simulink model "Solver"  (R2016b)
settings: Solver=ode4  StartTime=0.0  StopTime=Inf  FixedStep=base_dT  RelTol=1e-3
values from neighbouring files (symbols this model uses):
  base_dT = Simulink.Parameter    [SolverInit.m]
  E2C_bEgoFol = Simulink.Parameter    [SolverInit.m]
  E2C_bUseCollo = Simulink.Parameter    [SolverInit.m]
  E2C_c2_dTB = Simulink.Parameter    [SolverInit.m]
  E2C_c_dTB = Simulink.Parameter    [SolverInit.m]
  E2C_d_HDW1 = Simulink.Parameter    [SolverInit.m]
  E2C_d_HDW2 = Simulink.Parameter    [SolverInit.m]
  E2C_DeltaT = Simulink.Parameter    [SolverInit.m]
  E2C_df_term = Simulink.Parameter    [SolverInit.m]
  E2C_dz_term = Simulink.Parameter    [SolverInit.m]
  E2C_Max_iter = Simulink.Parameter    [SolverInit.m]
  E2C_t_HDW1 = Simulink.Parameter    [SolverInit.m]
  E2C_t_HDW2 = Simulink.Parameter    [SolverInit.m]
  E2C_T_TB_thr = Simulink.Parameter    [SolverInit.m]
  E2C_tiSolverPeriod_C = Simulink.Parameter    [SolverInit.m]
  E2C_U_max = Simulink.Parameter    [SolverInit.m]
  E2C_U_min = Simulink.Parameter    [SolverInit.m]
  E2C_V_max = Simulink.Parameter    [SolverInit.m]
  E2C_V_min = Simulink.Parameter    [SolverInit.m]
  E2C_w_delta_u = Simulink.Parameter    [SolverInit.m]
  E2C_w_epsilon_lin = Simulink.Parameter    [SolverInit.m]
  E2C_weight_TTB = Simulink.Parameter    [SolverInit.m]
  Inp_mf_exh_par = Simulink.Parameter    [SolverInit.m]
  Inp_t_eu_par = Simulink.Parameter    [SolverInit.m]
  NP_trial = Simulink.Parameter    [SolverInit.m]
  t_EndSimulation = Simulink.Parameter    [SolverInit.m]
  t_StartSimulation = Simulink.Parameter    [SolverInit.m]
libraries: simulink x3, dspsigops x2
(part 1 of 2)
settings Model: Creator=Tulga Ersal  LastModifiedBy=Hcn
settings OptimizationCC: BlockReduction=off  BooleanDataType=off  LifeSpan=inf
settings DebuggingCC: SaveWithParameterizedLinksMsg=none  UnderspecifiedInitializationDetection=Classic  MergeDetectMultiDrivingBlocksExec=none  SignalResolutionControl=TryResolveAllWithWarning  SFUnexpectedBacktrackingDiag=warning  SFNoUnconditionalDefaultTransitionDiag=warning  SFExecutionAtInitializationDiag=none
settings HardwareCC: TargetBitPerPointer=64  TargetBitPerSizeT=64  TargetBitPerPtrDiffT=64  TargetLongLongMode=on  TargetIntDivRoundTo=Zero  TargetEndianess=LittleEndian  TargetWordSize=64  TargetHWDeviceType=MATLAB Host  ProdEqTarget=off
settings ModelReferenceCC: PropagateSignalLabelsOutOfModel=off
settings GRTTargetCC: TargetLangStandard=C89/C90 (ANSI)
settings ConfigComp: CovMetricSettings=dw  CovHtmlReporting=on  CovSaveCumulativeToWorkspaceVar=on  CovSaveSingleToWorkspaceVar=on  CovExternalEMLEnable=off

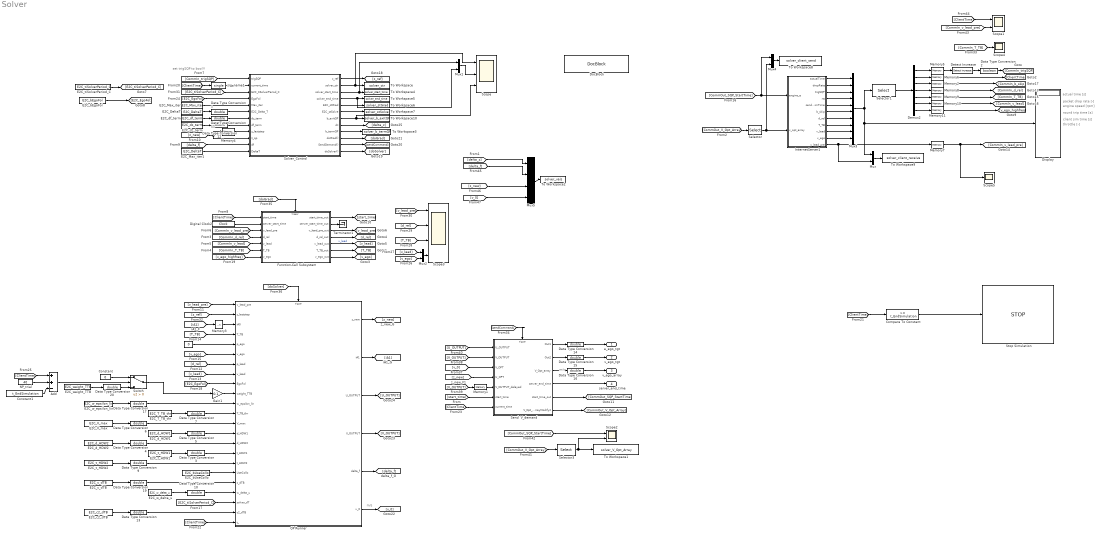
== system Solver ==
  note: set trigSQP to bool!!
  note: packet drop rate [-]
  note: actual time [s]
  note: engine speed [rpm]
  note: round trip time [s]
  note: client sim time [s]
  note: throttle [-]
  note: m/s
  note: m/s
  "\t" : Constant  Value=0
  Add : Sum  Inputs=++-
  Compare To Constant : simulink/Logic and Bit Operations/Compare To Constant  relop=>=  const=t_EndSimulation  OutDataTypeStr=boolean
  Constant : Constant  Value=0
  Constant1 : Constant  Value=t_EndSimulation
  Data Type Conversion{1,3..7,9..17,19..20} (17 alike) : DataTypeConversion  OutDataTypeStr=double
  Data Type Conversion2 : DataTypeConversion  OutDataTypeStr=boolean
  Demux2 : Demux  Outputs=7
  Detect Increase : simulink/Logic and Bit Operations/Detect Increase  vinit=0.0  OutDataTypeStr=boolean
  Digital Clock2 : DigitalClock  SampleTime=base_dT
  Display : Display
  DocBlock : simulink/Model-Wide Utilities/DocBlock  DocumentType=Text
      content=|
      | 110719T1200         -Finish chart for customized process control
      | 110719T1500         -use Ts=0.1(hardcoded), run server model alone, process control works with EgoFol=1.
      | 110719T1630         -use Ts=base_dT=0.01, run server & client. EgoFol=1.
      | 111119T1200         -Use last_v_opt(solver_start-delayed(solver_start) ) as current v_ego_tgt.
      |                     -Put the modification in Send V_demand subsys.
      |                     -Avoid using another block with detectchange in solver_end_time to trigger this modification.
      |                     -Clean the model and setup communication input/output ports (magenta)
      |                     -Modify Solver_Control so that EgoFol=0 case also works
      | 111119T2200         -Comment out "simulink execution control"
      |                     -If at one step "solver_exec_time>1s", the delay will cumulate
      |                     -need logic control in client to decide whether to skip a trigger.
      | 111219T1300         -Use Client time to set b_termQP.
      |                     -Set E2C_DeltaT=0.3s, save 0.3s for communication
      |                     -Cannot reset if one communication takes long time.
      | Client_112619T1415  -Created from PlatoonModel_Chunan_2016b_112119T1155 and InternetClient_112619T1300.
      |                     -Contains the whole vehicle model.
      |                     -Set up memory for CommOut_V_Opt_Array to align change for CommOut_V_Opt_Array and Comm_Start_Time.
      | Solver_112619T1415  -Created.
      |                     -Add semicolon in state flow to avoid printing intermediate variables.
      | Solver_112719T1142  -Add solver_ctr to workspace
      |                     -Do 10 "dosolver" in 1 step to compensate for base_dT=0.1s. If base_dT=0.01, use 1 dosolver.
      | Solver_112719T2200  -PlatoonModel_Chunan_2016b_112719T2200_solver/Send  V_demand/Triggered Subsystem.
      |                     Change also ceil(current_time-last_start_time).
      | C/S_122019T1424     -Add to resolve rtt issue. Not very useful on full model.:
      |                             while (myIns.simTime > timeNow*1)
      |                          {
      |                              QueryPerformanceCounter(&LItNow);
      |                              timeNow = ((double)(LItNow.QuadPart - G.LIstartTime.QuadPart)) / ((double)(G.LIticksPerSecond.QuadPart)) ;
      |                          }
      | C+S_122019T1618     -Put original solver and client into one system.
      |                     -Now the sent information are place holders to maintain dimension.
      |                     -Finally if this works, the client will be BBK and only sends
      |                     torque, TTB. Solver sends Ne, Alpha.
      | S_122819T1229 (C_122019T1618)
      |                     -Apply changes from Tulga in email "reducing delay further" to 122019T1618.
      |                     -rrt maintains to be 0.02s = base_dT.
      | S_122819T1301 (C_122019T1424)
      |                     -Apply changes from Tulga in email "reducing delay further" to 122019T1424.
      |                     -rrt drops to 0.02s = base_dT.
      |                     -But optimization result is still bad.
      |                     Does not recover optimal results similar to platoonmodel(without interenet),
      |                     like in version S_122819T1229.
      |                     -(!!!)switch Commin_v_lead and v_ego_highfreq at output of InternetServer1 demux.
      | %%%%%%%%%%%%%%%%%%%%%%%%%%%%%%%%%%%%%%%%%%%%%%%%%%%%%%%%%%%%%%%%%%%%%%%%%%
      | %                        3-computer setup                                %
      | %%%%%%%%%%%%%%%%%%%%%%%%%%%%%%%%%%%%%%%%%%%%%%%%%%%%%%%%%%%%%%%%%%%%%%%%%%
      | Solver_01022020T1343
      |                     -Create "InternetSolverInit.m" file for initialization.
      |                     -Only need "SpeedAcceMap8.mat" as external datasource.
  E2C_DeltaT : Constant  Value=E2C_DeltaT  OutDataTypeStr=double
  E2C_Max_iter : Constant  Value=E2C_Max_iter  OutDataTypeStr=int8
  E2C_Max_iter1 : Constant  Value=E2C_DeltaT  OutDataTypeStr=single
  E2C_T_TB_thr : Constant  Value=E2C_T_TB_thr  OutDataTypeStr=double
  E2C_V_max : Constant  Value=E2C_V_max  OutDataTypeStr=double
  E2C_bEgoFol : Constant  Value=E2C_bEgoFol  OutDataTypeStr=boolean
  E2C_bUseCollo : Constant  Value=E2C_bUseCollo  OutDataTypeStr=boolean
  E2C_c2_dTB : Constant  Value=E2C_c2_dTB  OutDataTypeStr=double
  E2C_c_dTB : Constant  Value=E2C_c_dTB  OutDataTypeStr=double
  E2C_d_HDW1 : Constant  Value=E2C_d_HDW1  OutDataTypeStr=double
  E2C_d_HDW2 : Constant  Value=E2C_d_HDW2  OutDataTypeStr=double
  E2C_df_term : Constant  Value=E2C_df_term  OutDataTypeStr=double
  E2C_dz_term : Constant  Value=E2C_dz_term  OutDataTypeStr=double
  E2C_t_HDW1 : Constant  Value=E2C_t_HDW1  OutDataTypeStr=double
  E2C_t_HDW2 : Constant  Value=E2C_t_HDW2  OutDataTypeStr=double
  E2C_tiSolverPeriod_C : Constant  Value=E2C_tiSolverPeriod_C  OutDataTypeStr=single
  E2C_w_delta_u : Constant  Value=E2C_w_delta_u  OutDataTypeStr=double
  E2C_w_epsilon_lin : Constant  Value=E2C_w_epsilon_lin  OutDataTypeStr=double
  E2C_weight_TTB : Constant  Value=E2C_weight_TTB  OutDataTypeStr=double
  Function-Call Subsystem : Subsystem  TreatAsAtomicUnit=on
  Gain1 : Gain  Gain=0.1
  InternetServer1 : Subsystem  mask(20-sim 4.6 S-Function block){}
      mask help:
      | This block is generated by the 20-sim Matlab Code Generator.
      |
      | * look under the mask to get information on the ports
      | * press Help for more detailed information
      | * the parameters of this block are:
      mask Help:
      | This block is generated by the 20-sim Matlab Code Generator<br>
      | The block parameters are:<br><blockquote></blockquote>
      | Generated at:<br>
      | <blockquote><b>date:  </b>June 14, 2017<br>
      | <b>time:  </b>4:16:43 PM<br></blockquote>
      | From the following 20-sim model:<br>
      | <blockquote><b>submodel:  </b>InternetServer<br>
      | <b>model:  </b>export to Simulink - UM<br>
      | <b>file:  </b>C:\Users\Tulga Ersal\Desktop\For Xueru\export to Simulink - UM.emx<br>
      | <b>experiment:  </b>C:\Users\Tulga Ersal\Desktop\For Xueru\export to Simulink - UM.emx<br></blockquote>
      | Using the following 20-sim license:<br>
      | <blockquote><b>user:  </b>The University of Michigan<br>
      | <b>from:  </b>20-sim 4.6 Student License<br>
      | <b>build: </b>4.6.1.6898<br></blockquote>
  Memory1 : Memory  InheritSampleTime=on  LinearizeAsDelay=on
  Memory{2,5..6,10..11} (5 alike) : Memory
  Memory3 : Memory  X0=false(4*40+2*40+2,1)  InheritSampleTime=on  LinearizeAsDelay=on
  Memory4 : Memory  X0=zeros(41, 1)  InheritSampleTime=on  LinearizeAsDelay=on
  Memory7 : Memory  X0=zeros(40,1)  InheritSampleTime=on  LinearizeAsDelay=on
  Memory8 : Memory  X0=10
  Memory9 : Memory  X0=200
  Mux{,1..2,4} (4 alike) : Mux  Inputs=2
  Mux3 : Mux  Inputs=10
  Mux5 : Mux
  NP_trial : Constant  Value=40
  QP Runner : Subsystem  TreatAsAtomicUnit=on
  Scope : Scope  NumInputPorts=3
  Scope1 : Scope  NumInputPorts=2
  Scope2 : Scope  NumInputPorts=2
  Scope3 : Scope  NumInputPorts=4
  Scope4 : Scope
  Scope5 : Scope
  Selector : Selector  InputPortWidth=40  IndexOptions=Index vector (dialog)  Indices=[1:40]  OutputSizes=1
  Selector1 : Selector  InputPortWidth=10  IndexOptions=Index vector (dialog)  Indices=[3,5,6,7,8,9,10]  OutputSizes=1
  Selector3 : Selector  InputPortWidth=40  IndexOptions=Index vector (dialog)  Indices=[1:10]  OutputSizes=1
  Send  V_demand : Subsystem  TreatAsAtomicUnit=on
  Solver_Control : Stateflow chart  TreatAsAtomicUnit=on
  Stop Simulation : Stop
  Switch : Switch  Criteria=u2 > Threshold
  Terminator1 : Terminator
  To Workspace : ToWorkspace  VariableName=solver_ctr  SaveFormat=Timeseries  SampleTime=-1
  To Workspace1 : ToWorkspace  VariableName=solver_V_Opt_Array  SaveFormat=Timeseries  SampleTime=-1
  To Workspace10 : ToWorkspace  VariableName=solver_b_exitQP  SaveFormat=Timeseries  SampleTime=-1
  To Workspace2 : ToWorkspace  VariableName=solver_vals  SaveFormat=Timeseries  SampleTime=-1
  To Workspace3 : ToWorkspace  VariableName=solver_b_termQP  SaveFormat=Timeseries  SampleTime=-1
  To Workspace4 : ToWorkspace  VariableName=solver_start_time  SaveFormat=Timeseries  SampleTime=-1
  To Workspace5 : ToWorkspace  VariableName=solver_end_time  SaveFormat=Timeseries  SampleTime=-1
  To Workspace6 : ToWorkspace  VariableName=solver_stGrad  SaveFormat=Timeseries  SampleTime=-1
  To Workspace7 : ToWorkspace  VariableName=solver_stSolve  SaveFormat=Timeseries  SampleTime=-1
  To Workspace8 : ToWorkspace  VariableName=solver_client_send  SaveFormat=Timeseries  SampleTime=-1
  To Workspace9 : ToWorkspace  VariableName=solver_client_receive  SaveFormat=Timeseries  SampleTime=-1
  sig_name1 : DataTypeConversion  OutDataTypeStr=single
  a_ego_tgt : Outport
  v_ego_tgt : Outport  Port=2
  v_ego_array : Outport  Port=3  InitialOutput=zeros(40,1)
  server_end_time : Outport  Port=4  InitialOutput=0
  wires:
  Demux2/1 -> Memory5/1
  Demux2/3 -> Memory2/1
  Demux2/2 -> Memory6/1
  [ClientTime] -> Function-Call Subsystem/1(start_time)
  Digital Clock2/1 -> Function-Call Subsystem/2(server_start_time)
  [ClientTime] -> sig_name1/1
  E2C_tiSolverPeriod_C/1 -> [E2C_tiSolverPeriod_C]
  sig_name1/1 -> Solver_Control/2(current_time)
  Data Type Conversion12/1 -> Solver_Control/8(df_term)
  E2C_df_term/1 -> Data Type Conversion11/1
  Data Type Conversion11/1 -> Solver_Control/7(dz_term)
  E2C_dz_term/1 -> Data Type Conversion12/1
  E2C_bEgoFol/1 -> [E2C_EgoFol]
  Data Type Conversion1/1 -> Solver_Control/6(E2C_Delta_T)
  E2C_DeltaT/1 -> Data Type Conversion1/1
  E2C_Max_iter/1 -> Solver_Control/5(Max_iter)
  [CommIn_trigSQP] -> Solver_Control/1(trigSQP)
  [T_TB] -> QP Runner/4(T_TB)
  [v_lead] -> QP Runner/8(v_lead)
  [d_rel] -> QP Runner/7(p_lead)
  QP Runner/1(z_new) -> [z_new]
  Memory3/1 -> QP Runner/3(iA0)
  QP Runner/3(U_OUTPUT) -> [U_OUTPUT]
  QP Runner/4(V_OUTPUT) -> [V_OUTPUT]
  [v_lead_pre] -> QP Runner/1(v_lead_pre)
  Data Type Conversion15/1 -> v_ego_tgt/1
  Send  V_demand/1(Out1) -> Data Type Conversion14/1
  [v_ego] -> QP Runner/6("v_ego ")
  QP Runner/6(v_0) -> [v_0]
  Gain1/1 -> QP Runner/10(weight_TTB)
  Data Type Conversion17/1 -> QP Runner/11(w_epsilon_lin)
  Data Type Conversion7/1 -> QP Runner/12(T_TB_thr)
  "\t"/1 -> QP Runner/5(p_ego)
  Data Type Conversion6/1 -> QP Runner/13(V_max)
  Data Type Conversion5/1 -> QP Runner/14(d_HDW1)
  Data Type Conversion4/1 -> QP Runner/15(d_HDW2)
  Data Type Conversion9/1 -> QP Runner/17(t_HDW2)
  Data Type Conversion3/1 -> QP Runner/16(t_HDW1)
  E2C_bUseCollo/1 -> QP Runner/18(UseCollo)
  E2C_c_dTB/1 -> Data Type Conversion19/1
  Data Type Conversion10/1 -> QP Runner/20(w_delta_u)
  E2C_t_HDW2/1 -> Data Type Conversion9/1
  [z_new] -> Send  V_demand/4(U_OPT)
  QP Runner/5(delta_f) -> [delta_f]
  QP Runner/2(iA1) -> [iA1]
  [iA1] -> Memory3/1
  E2C_t_HDW1/1 -> Data Type Conversion3/1
  E2C_d_HDW2/1 -> Data Type Conversion4/1
  E2C_d_HDW1/1 -> Data Type Conversion5/1
  E2C_V_max/1 -> Data Type Conversion6/1
  E2C_T_TB_thr/1 -> Data Type Conversion7/1
  E2C_w_epsilon_lin/1 -> Data Type Conversion17/1
  Switch/1 -> Gain1/1
  Data Type Conversion19/1 -> QP Runner/19("c_dTB ")
  E2C_w_delta_u/1 -> Data Type Conversion10/1
  [E2C_tiSolverPeriod_C] -> QP Runner/21(solver_dT)
  Data Type Conversion13/1 -> QP Runner/22(c2_dTB)
  E2C_c2_dTB/1 -> Data Type Conversion13/1
  Send  V_demand/3(V_Opt_array) -> Data Type Conversion16/1
  [doSolver] -> QP Runner/Trigger
  Memory1/1 -> Send  V_demand/5(V_OUTPUT_delayed)
  [sendCommand] -> Send  V_demand/Trigger
  Send  V_demand/4(server_end_time) -> server_end_time/1
  Data Type Conversion14/1 -> a_ego_tgt/1
  Send  V_demand/2(Out2) -> Data Type Conversion15/1
  Data Type Conversion16/1 -> v_ego_array/1
  [delta_f] -> Solver_Control/11(df)
  [z_new] -> Solver_Control/10(z_qp), Memory4/1
  Memory4/1 -> Solver_Control/9(z_laststep)
  [E2C_EgoFol] -> QP Runner/9(EgoFol)
  Solver_Control/10(doGrad()) -> [doGrad]
  Function-Call Subsystem/6(T_TB_out) -> [T_TB]
  Function-Call Subsystem/5(v_lead_out) -> [v_lead]  "v_lead"
  Function-Call Subsystem/4(d_rel_out) -> [d_rel]
  Function-Call Subsystem/3(v_lead_pre_out) -> [v_lead_pre]
  Function-Call Subsystem/7(v_ego_out) -> [v_ego]
  [v_ego_highfreq] -> Function-Call Subsystem/7(v_ego)
  Data Type Conversion2/1 -> [CommIn_trigSQP]
  Memory5/1 -> Detect Increase/1
  Send  V_demand/5(start_time_out) -> [CommOut_SQP_StartTime]
  Detect Increase/1 -> Data Type Conversion2/1
  Function-Call Subsystem/1(start_time_out) -> [start_time]
  [start_time] -> Send  V_demand/6(start_time)
  Send  V_demand/6(V_Opt_ArrayModify2) -> [CommOut_V_Opt_Array]
  E2C_Max_iter1/1 -> Solver_Control/12(DeltaT)
  Demux2/4 -> Memory8/1
  [CommIn_d_rel] -> Function-Call Subsystem/4(d_rel)
  [CommIn_v_lead] -> Function-Call Subsystem/5(v_lead)
  [CommIn_T_TB] -> Function-Call Subsystem/6(T_TB)
  [CommIn_v_lead_pre] -> Function-Call Subsystem/3(v_lead_pre)
  Memory6/1 -> [ClientTime]
  InternetServer1/3(trigSQP) -> Mux3/3
  InternetServer1/4(rtt) -> Mux3/4
  InternetServer1/2(dropRate) -> Mux3/2
  InternetServer1/5(sendSimTime) -> Mux3/5
  InternetServer1/1(actualTime) -> Mux3/1
  InternetServer1/6(b_skip) -> Mux3/6
  Mux3/1 -> Display/1, Mux/1, Selector1/1
  InternetServer1/7(d_rel) -> Mux3/7
  InternetServer1/8(T_TB) -> Mux3/8
  InternetServer1/9(v_lead) -> Mux3/9
  InternetServer1/10(v_ego) -> Mux3/10
  InternetServer1/11(v_lead_pre) -> Mux/2, Memory7/1
  [CommOut_V_Opt_Array] -> Selector/1
  [CommOut_SQP_StartTime] -> InternetServer1/1(engine_e), Mux4/1
  Memory7/1 -> Scope5/1, [CommIn_v_lead_pre]
  Selector1/1 -> Demux2/1
  Demux2/5 -> Memory9/1
  Demux2/6 -> Memory10/1
  Demux2/7 -> Memory11/1
  Memory8/1 -> [CommIn_d_rel]
  Memory9/1 -> [CommIn_T_TB]
  Memory10/1 -> [CommIn_v_lead]
  Memory11/1 -> [v_ego_highfreq]
  [ClientTime] -> Compare To Constant/1
  Compare To Constant/1 -> Stop Simulation/1
  Selector3/1 -> Scope2/2, To Workspace1/1
  [ClientTime] -> QP Runner/23(t_)
  Solver_Control/2(solver_ctr) -> Scope/1, To Workspace/1
  [ClientTime] -> Send  V_demand/7(current_time)
  Solver_Control/3(solver_start_time) -> Mux1/1, To Workspace4/1
  Solver_Control/4(solver_end_time) -> Mux1/2, To Workspace5/1
  Solver_Control/5(E2C_stGrad) -> To Workspace6/1
  Solver_Control/6(E2C_stSolve) -> To Workspace7/1
  E2C_weight_TTB/1 -> Data Type Conversion20/1
  [ClientTime] -> Add/1
  NP_trial/1 -> Add/2
  Constant1/1 -> Add/3
  Add/1 -> Switch/2
  Data Type Conversion20/1 -> Switch/3
  Constant/1 -> Switch/1
  Selector/1 -> Mux4/2, InternetServer1/2(v_opt_array)
  Mux1/1 -> Scope/2
  Solver_Control/7(b_exitQP) -> Scope/3, To Workspace10/1
  Mux2/1 -> Scope3/4
  Mux/1 -> To Workspace9/1
  Mux4/1 -> To Workspace8/1
  [v_ego] -> Mux2/2
  [v_lead] -> Mux2/1
  [T_TB] -> Scope3/3
  [d_rel] -> Scope3/2
  [v_lead_pre] -> Scope3/1
  Function-Call Subsystem/2(server_start_time_out) -> Terminator1/1
  [E2C_EgoFol] -> Solver_Control/4(EgoFol)
  [E2C_tiSolverPeriod_C] -> Solver_Control/3(E2C_tiSolverPeriod_C)
  Solver_Control/1(z_ref) -> [z_ref]
  [z_ref] -> QP Runner/2(z_laststep)
  [CommIn_T_TB] -> Scope4/1
  Solver_Control/12(doSolver()) -> [doSolver]
  Solver_Control/11(SendDemand()) -> [sendCommand]
  [doGrad] -> Function-Call Subsystem/Trigger
  [v_0] -> Send  V_demand/3(V_OPT)
  [V_OUTPUT] -> Send  V_demand/2(V_OUTPUT)
  [V_OUTPUT] -> Memory1/1
  [U_OUTPUT] -> Send  V_demand/1(U_OUTPUT)
  [CommOut_V_Opt_Array] -> Selector3/1
  [CommOut_SQP_StartTime] -> Scope2/1
  [ClientTime] -> Scope1/1
  [CommIn_v_lead_pre] -> Scope1/2
  Memory2/1 -> [CommIn_b_skip]
  Solver_Control/8(dz) -> [delta_z]
  [delta_f] -> Mux5/2
  [delta_z] -> Mux5/1
  Mux5/1 -> To Workspace2/1
  [z_new] -> Mux5/3
  [v_0] -> Mux5/4
  Solver_Control/9(b_termQP) -> To Workspace3/1

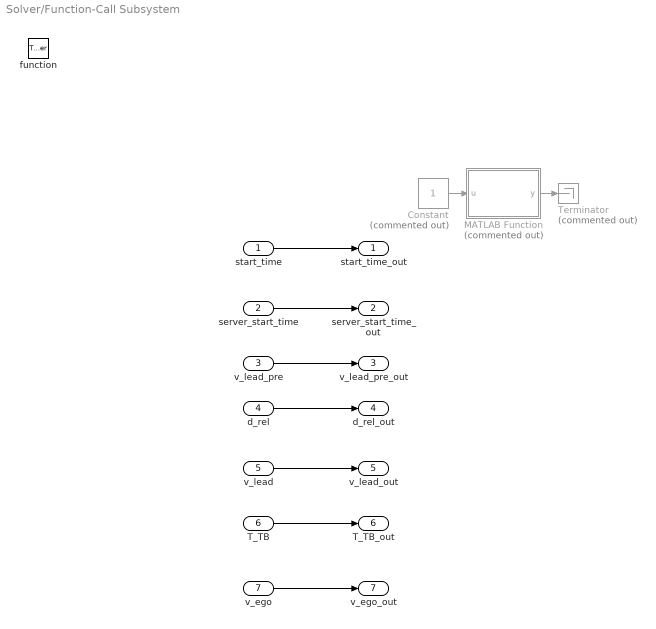
== system Solver/Function-Call Subsystem ==
  start_time : Inport
  server_start_time : Inport  Port=2
  v_lead_pre : Inport  Port=3
  d_rel : Inport  Port=4
  v_lead : Inport  Port=5
  T_TB : Inport  Port=6
  v_ego : Inport  Port=7
  function : TriggerPort  TriggerType=function-call  VariantControl=Variant
  Constant : Constant  Commented=on
  MATLAB Function : MATLAB Function  Commented=on  TreatAsAtomicUnit=on
  Terminator : Terminator  Commented=on
  start_time_out : Outport
  server_start_time_out : Outport  Port=2
  v_lead_pre_out : Outport  Port=3
  d_rel_out : Outport  Port=4
  v_lead_out : Outport  Port=5
  T_TB_out : Outport  Port=6
  v_ego_out : Outport  Port=7
  wires:
  start_time/1 -> start_time_out/1
  server_start_time/1 -> server_start_time_out/1
  v_lead_pre/1 -> v_lead_pre_out/1
  d_rel/1 -> d_rel_out/1
  v_lead/1 -> v_lead_out/1
  T_TB/1 -> T_TB_out/1
  Constant/1 -> MATLAB Function/1(u)
  MATLAB Function/1(y) -> Terminator/1
  v_ego/1 -> v_ego_out/1

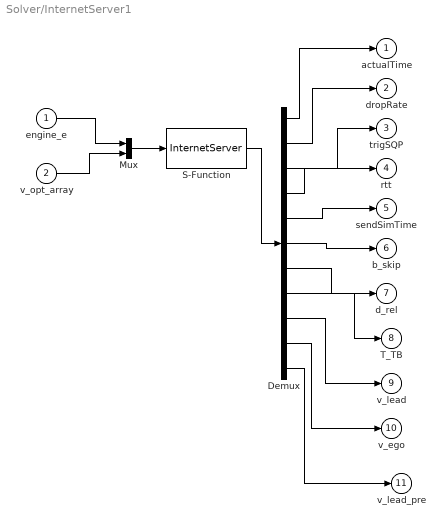
== system Solver/InternetServer1 ==
  engine_e : Inport
  v_opt_array : Inport  Port=2
  Demux : Demux  Outputs=[1 1 1 1 1 1 1 1 1 1 40]
  Mux : Mux  Inputs=[1 40 ]
  S-Function : S-Function  FunctionName=InternetServer  SFunctionDeploymentMode=off  EnableBusSupport=off
  actualTime : Outport
  dropRate : Outport  Port=2
  trigSQP : Outport  Port=3
  rtt : Outport  Port=4
  sendSimTime : Outport  Port=5
  b_skip : Outport  Port=6
  d_rel : Outport  Port=7
  T_TB : Outport  Port=8
  v_lead : Outport  Port=9
  v_ego : Outport  Port=10
  v_lead_pre : Outport  Port=11
  wires:
  engine_e/1 -> Mux/1
  Demux/1 -> actualTime/1
  Demux/2 -> dropRate/1
  Demux/3 -> trigSQP/1
  Demux/4 -> rtt/1
  Demux/5 -> sendSimTime/1
  Demux/6 -> b_skip/1
  Mux/1 -> S-Function/1
  S-Function/1 -> Demux/1
  Demux/7 -> d_rel/1
  Demux/8 -> T_TB/1
  Demux/9 -> v_lead/1
  Demux/10 -> v_ego/1
  Demux/11 -> v_lead_pre/1
  v_opt_array/1 -> Mux/2

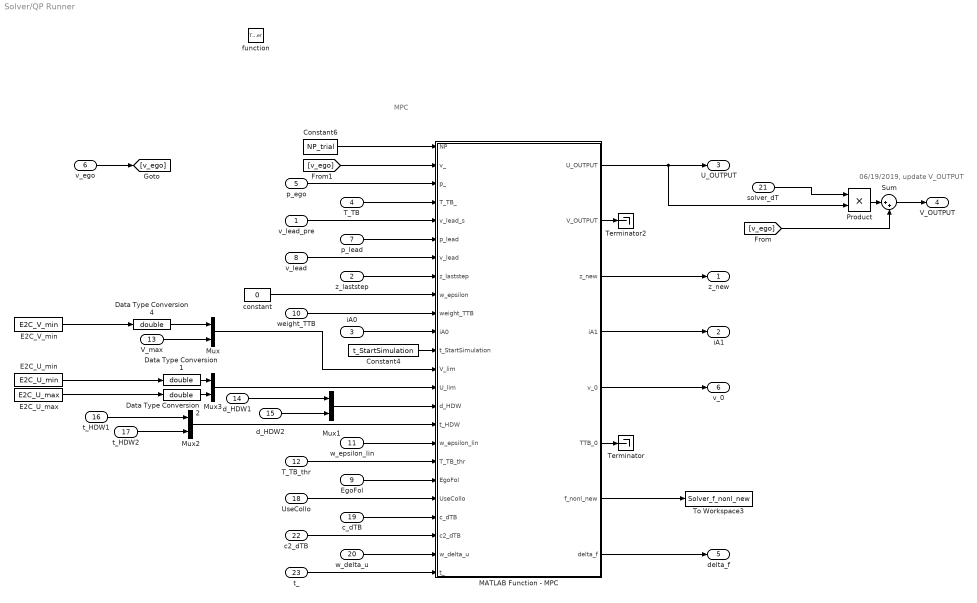
== system Solver/QP Runner ==
  note: 06/19/2019, update V_OUTPUT
  note: MPC
  v_lead_pre : Inport
  z_laststep : Inport  Port=2
  iA0 : Inport  Port=3
  T_TB : Inport  Port=4
  p_ego : Inport  Port=5
  "v_ego " : Inport  Port=6
  p_lead : Inport  Port=7
  v_lead : Inport  Port=8
  EgoFol : Inport  Port=9
  weight_TTB : Inport  Port=10
  w_epsilon_lin : Inport  Port=11
  T_TB_thr : Inport  Port=12
  V_max : Inport  Port=13
  d_HDW1 : Inport  Port=14
  d_HDW2 : Inport  Port=15
  t_HDW1 : Inport  Port=16
  t_HDW2 : Inport  Port=17
  UseCollo : Inport  Port=18
  "c_dTB " : Inport  Port=19
  w_delta_u : Inport  Port=20
  solver_dT : Inport  Port=21
  c2_dTB : Inport  Port=22
  t_ : Inport  Port=23
  function : TriggerPort  TriggerType=function-call  VariantControl=Variant
  Constant4 : Constant  Value=t_StartSimulation
  Constant6 : Constant  Value=NP_trial
  Data Type Conversion1 : DataTypeConversion  OutDataTypeStr=double
  Data Type Conversion2 : DataTypeConversion  OutDataTypeStr=double
  Data Type Conversion4 : DataTypeConversion  OutDataTypeStr=double
  E2C_U_max : Constant  Value=E2C_U_max  OutDataTypeStr=single
  E2C_U_min : Constant  Value=E2C_U_min  OutDataTypeStr=single
  E2C_V_min : Constant  Value=E2C_V_min  OutDataTypeStr=single
  MATLAB Function - MPC : MATLAB Function  TreatAsAtomicUnit=on
  Mux{,1..3} (4 alike) : Mux  Inputs=2
  Product : Product
  Sum : Sum  Inputs=|++
  Terminator : Terminator
  Terminator2 : Terminator
  To Workspace3 : ToWorkspace  VariableName=Solver_f_nonl_new  SaveFormat=Timeseries  SampleTime=-1
  constant : Constant  Value=0  OutDataTypeStr=Inherit: Inherit via back propagation
  z_new : Outport  InitialOutput=zeros(41,1)
  iA1 : Outport  Port=2  InitialOutput=zeros(242,1)
  U_OUTPUT : Outport  Port=3  InitialOutput=0
  V_OUTPUT : Outport  Port=4  InitialOutput=0
  delta_f : Outport  Port=5  InitialOutput=zeros(1,1)
  v_0 : Outport  Port=6  InitialOutput=zeros(40,1)
  wires:
  T_TB/1 -> MATLAB Function - MPC/4(T_TB_)
  p_ego/1 -> MATLAB Function - MPC/3(p_)
  v_lead/1 -> MATLAB Function - MPC/7(v_lead)
  v_lead_pre/1 -> MATLAB Function - MPC/5(v_lead_s)
  constant/1 -> MATLAB Function - MPC/9(w_epsilon)
  weight_TTB/1 -> MATLAB Function - MPC/10(weight_TTB)
  Constant6/1 -> MATLAB Function - MPC/1(NP)
  MATLAB Function - MPC/1(U_OUTPUT) -> U_OUTPUT/1, Product/2
  Sum/1 -> V_OUTPUT/1
  MATLAB Function - MPC/3(z_new) -> z_new/1
  z_laststep/1 -> MATLAB Function - MPC/8(z_laststep)
  MATLAB Function - MPC/4(iA1) -> iA1/1
  iA0/1 -> MATLAB Function - MPC/11(iA0)
  MATLAB Function - MPC/8(delta_f) -> delta_f/1
  Constant4/1 -> MATLAB Function - MPC/12(t_StartSimulation)
  Mux/1 -> MATLAB Function - MPC/13(V_lim)
  Mux3/1 -> MATLAB Function - MPC/14(U_lim)
  Mux1/1 -> MATLAB Function - MPC/15(d_HDW)
  Mux2/1 -> MATLAB Function - MPC/16(t_HDW)
  w_epsilon_lin/1 -> MATLAB Function - MPC/17(w_epsilon_lin)
  T_TB_thr/1 -> MATLAB Function - MPC/18(T_TB_thr)
  MATLAB Function - MPC/5(v_0) -> v_0/1
  EgoFol/1 -> MATLAB Function - MPC/19(EgoFol)
  MATLAB Function - MPC/6(TTB_0) -> Terminator/1
  MATLAB Function - MPC/7(f_nonl_new) -> To Workspace3/1
  p_lead/1 -> MATLAB Function - MPC/6(p_lead)
  Data Type Conversion4/1 -> Mux/1
  V_max/1 -> Mux/2
  d_HDW1/1 -> Mux1/1
  d_HDW2/1 -> Mux1/2
  t_HDW1/1 -> Mux2/1
  t_HDW2/1 -> Mux2/2
  UseCollo/1 -> MATLAB Function - MPC/20(UseCollo)
  "c_dTB "/1 -> MATLAB Function - MPC/21(c_dTB)
  w_delta_u/1 -> MATLAB Function - MPC/23(w_delta_u)
  Product/1 -> Sum/1
  solver_dT/1 -> Product/1
  MATLAB Function - MPC/2(V_OUTPUT) -> Terminator2/1
  c2_dTB/1 -> MATLAB Function - MPC/22(c2_dTB)
  E2C_V_min/1 -> Data Type Conversion4/1
  E2C_U_max/1 -> Data Type Conversion2/1
  E2C_U_min/1 -> Data Type Conversion1/1
  Data Type Conversion1/1 -> Mux3/1
  Data Type Conversion2/1 -> Mux3/2
  t_/1 -> MATLAB Function - MPC/24(t_)
  [v_ego] -> Sum/2
  "v_ego "/1 -> [v_ego]
  [v_ego] -> MATLAB Function - MPC/2(v_)

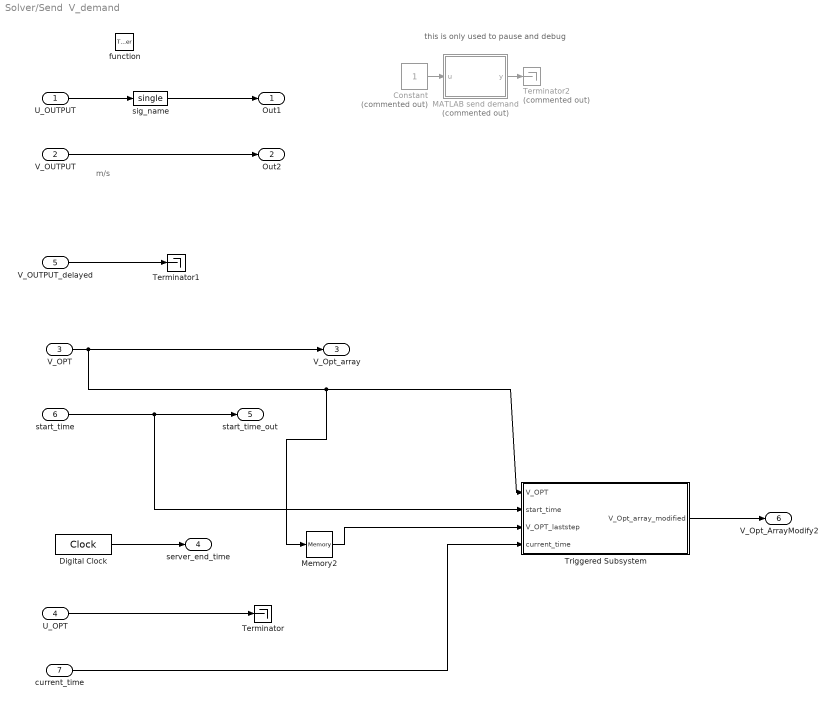
== system Solver/Send  V_demand ==
  note: this is only used to pause and debug
  note: m/s
  U_OUTPUT : Inport
  V_OUTPUT : Inport  Port=2
  V_OPT : Inport  Port=3
  U_OPT : Inport  Port=4
  V_OUTPUT_delayed : Inport  Port=5
  start_time : Inport  Port=6
  current_time : Inport  Port=7
  function : TriggerPort  TriggerType=function-call  VariantControl=Variant
  Constant : Constant  Commented=on
  Digital Clock : DigitalClock  SampleTime=-1
  MATLAB send demand : MATLAB Function  Commented=on  TreatAsAtomicUnit=on
  Memory2 : Memory  X0=zeros(40,1)  InheritSampleTime=on  LinearizeAsDelay=on
  Terminator : Terminator
  Terminator1 : Terminator
  Terminator2 : Terminator  Commented=on
  Triggered Subsystem : Subsystem  TreatAsAtomicUnit=on
  sig_name : DataTypeConversion  OutDataTypeStr=single
  Out1 : Outport  InitialOutput=0
  Out2 : Outport  Port=2  InitialOutput=0
  V_Opt_array : Outport  Port=3  InitialOutput=zeros(40,1)
  server_end_time : Outport  Port=4  InitialOutput=0
  start_time_out : Outport  Port=5
  V_Opt_ArrayModify2 : Outport  Port=6
  wires:
  U_OUTPUT/1 -> sig_name/1
  U_OPT/1 -> Terminator/1
  sig_name/1 -> Out1/1
  V_OUTPUT/1 -> Out2/1
  V_OPT/1 -> V_Opt_array/1, Memory2/1, Triggered Subsystem/1(V_OPT)
  Digital Clock/1 -> server_end_time/1
  Constant/1 -> MATLAB send demand/1(u)
  MATLAB send demand/1(y) -> Terminator2/1
  Memory2/1 -> Triggered Subsystem/3(V_OPT_laststep)
  start_time/1 -> Triggered Subsystem/2(start_time), start_time_out/1
  Triggered Subsystem/1(V_Opt_array_modified) -> V_Opt_ArrayModify2/1
  V_OUTPUT_delayed/1 -> Terminator1/1
  current_time/1 -> Triggered Subsystem/4(current_time)

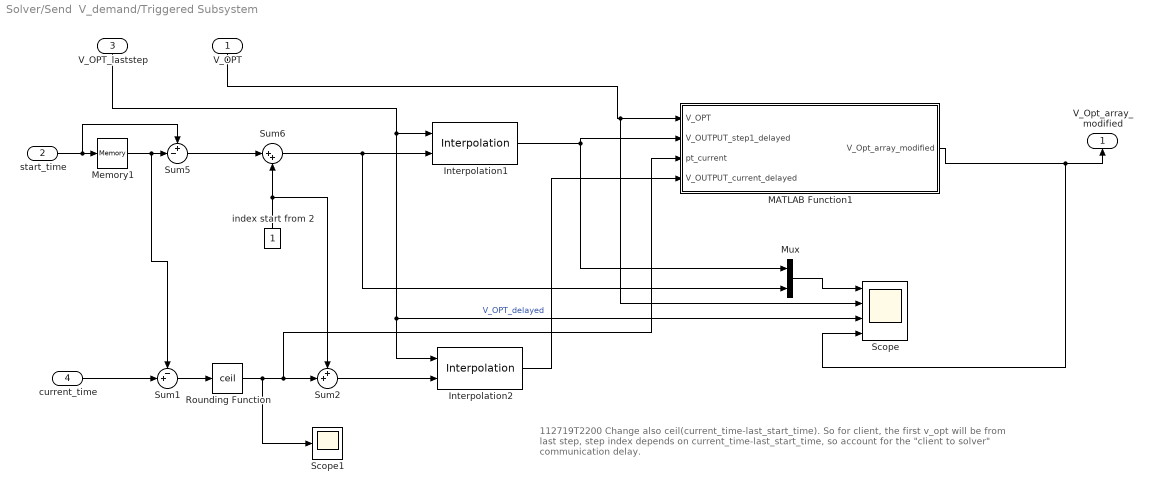
== system Solver/Send  V_demand/Triggered Subsystem ==
  note: 112719T2200
      | Change also ceil(current_time-last_start_time). So for client, the first v_opt
      | will be from last step, step index depends on current_time-last_start_time, so
      | account for the "client to solver" communication delay.
  V_OPT : Inport
  start_time : Inport  Port=2
  V_OPT_laststep : Inport  Port=3
  current_time : Inport  Port=4
  Interpolation1 : dspsigops/Interpolation  InterpSource=Input port  InterpPoints=[1.1 4.8 2.67 1.6 3.2]'  InterpMode=Linear  InterpL=3  InterpR=3  InterpAlpha=0.5  InvalidMode=Clip
  Interpolation2 : dspsigops/Interpolation  InterpSource=Input port  InterpPoints=[1.1 4.8 2.67 1.6 3.2]'  InterpMode=Linear  InterpL=3  InterpR=3  InterpAlpha=0.5  InvalidMode=Clip
  MATLAB Function1 : MATLAB Function  TreatAsAtomicUnit=on
  Memory1 : Memory  InheritSampleTime=on  LinearizeAsDelay=on
  Mux : Mux  Inputs=2
  Rounding Function : Rounding  Operator=ceil
  Scope : Scope  NumInputPorts=4
  Scope1 : Scope
  Sum1 : Sum  Inputs=-+|
  Sum2 : Sum  Inputs=++|
  Sum5 : Sum  Inputs=+-|
  Sum6 : Sum  Inputs=|++
  index start from 2 : Constant  OutDataTypeStr=single
  V_Opt_array_modified : Outport
  wires:
  V_OPT/1 -> Scope/2, MATLAB Function1/1(V_OPT)
  Sum6/1 -> Mux/2, Interpolation1/2
  V_OPT_laststep/1 -> Interpolation2/1, Scope/3, Interpolation1/1  "V_OPT_delayed"
  MATLAB Function1/1(V_Opt_array_modified) -> Scope/4, V_Opt_array_modified/1
  Interpolation1/1 -> Mux/1, MATLAB Function1/2(V_OUTPUT_step1_delayed)
  index start from 2/1 -> Sum2/1, Sum6/2
  start_time/1 -> Memory1/1, Sum5/1
  Memory1/1 -> Sum1/1, Sum5/2
  Sum5/1 -> Sum6/1
  Mux/1 -> Scope/1
  current_time/1 -> Sum1/2
  Sum1/1 -> Rounding Function/1
  Interpolation2/1 -> MATLAB Function1/4(V_OUTPUT_current_delayed)
  Sum2/1 -> Interpolation2/2
  Rounding Function/1 -> Scope1/1, MATLAB Function1/3(pt_current), Sum2/2
